simulink model "testConvert2Polyblock"  (Simulink 7.4)
settings: Solver=ode45  StartTime=0.0  StopTime=10.0  RelTol=1e-3
undefined symbols (not defined in the file or in its folder): magnitude
libraries: BLOM_Lib x3
settings Model: Creator=Kyle  LastModifiedBy=Kyle

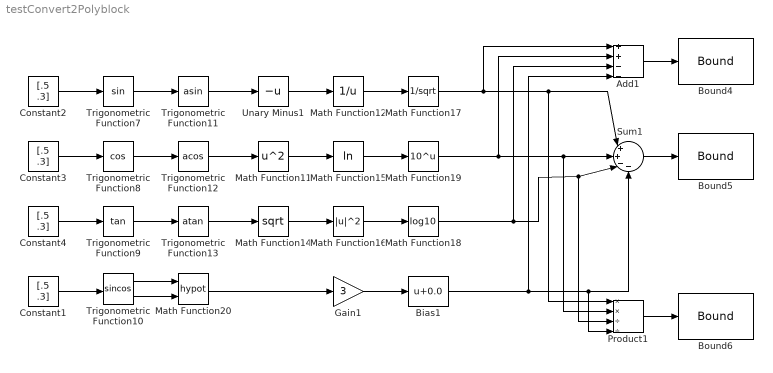
== system testConvert2Polyblock ==
  Add1 : Sum  Inputs=++--  OutDataType=fixdt(1, 16)  OutScaling=2^-10
  Bias1 : Bias  Bias=0.0
  Bound4 : BLOM_Lib/Bound  SystemSampleTime=-1  ub=6  lb=-6  initial_step=on  final_step=off  intermediate_step=off
  Bound5 : BLOM_Lib/Bound  SystemSampleTime=-1  ub=6  lb=-6  initial_step=off  final_step=off  intermediate_step=on
  Bound6 : BLOM_Lib/Bound  SystemSampleTime=-1  ub=6  lb=-6  initial_step=off  final_step=on  intermediate_step=off
  Constant{1..4} (4 alike) : Constant  Value=[.5 .3]  OutDataType=fixdt(1, 16)  OutScaling=2^0
  Gain1 : Gain  Gain=3  ParameterDataType=fixdt(1, 16)  ParameterScaling=2^0  OutDataType=fixdt(1, 16)  OutScaling=2^0
  Math Function11 : Math  Operator=square  OutDataType=fixdt(1, 16)  OutScaling=2^0  SaturateOnIntegerOverflow=on
  Math Function12 : Math  Operator=reciprocal  OutDataType=fixdt(1, 16)  OutScaling=2^0  SaturateOnIntegerOverflow=on
  Math Function14 : Math  Operator=sqrt  OutDataType=fixdt(1, 16)  OutScaling=2^0  SaturateOnIntegerOverflow=on
  Math Function15 : Math  Operator=log  OutDataType=fixdt(1, 16)  OutScaling=2^0  SaturateOnIntegerOverflow=on
  Math Function16 : Math  Operator=magnitude^2  OutDataType=fixdt(1, 16)  OutScaling=2^0  SaturateOnIntegerOverflow=on
  Math Function17 : Math  Operator=1/sqrt  OutDataType=fixdt(1, 16)  OutScaling=2^0  SaturateOnIntegerOverflow=on
  Math Function18 : Math  Operator=log10  OutDataType=fixdt(1, 16)  OutScaling=2^0  SaturateOnIntegerOverflow=on
  Math Function19 : Math  Operator=10^u  OutDataType=fixdt(1, 16)  OutScaling=2^0  SaturateOnIntegerOverflow=on
  Math Function20 : Math  Operator=hypot  OutDataType=fixdt(1, 16)  OutScaling=2^0  SaturateOnIntegerOverflow=on
  Product1 : Product  Inputs=**//  OutDataType=fixdt(1, 16)  OutScaling=2^0  RndMeth=Zero
  Sum1 : Sum  Inputs=|++--  OutDataType=fixdt(1, 16)  OutScaling=2^0
  Trigonometric Function10 : Trigonometry  Operator=sincos
  Trigonometric Function11 : Trigonometry  Operator=asin
  Trigonometric Function12 : Trigonometry  Operator=acos
  Trigonometric Function13 : Trigonometry  Operator=atan
  Trigonometric Function7 : Trigonometry
  Trigonometric Function8 : Trigonometry  Operator=cos
  Trigonometric Function9 : Trigonometry  Operator=tan
  Unary Minus1 : UnaryMinus
  wires:
  Constant2/1 -> Trigonometric Function7/1
  Constant3/1 -> Trigonometric Function8/1
  Constant4/1 -> Trigonometric Function9/1
  Constant1/1 -> Trigonometric Function10/1
  Trigonometric Function7/1 -> Trigonometric Function11/1
  Trigonometric Function8/1 -> Trigonometric Function12/1
  Trigonometric Function9/1 -> Trigonometric Function13/1
  Trigonometric Function11/1 -> Unary Minus1/1
  Trigonometric Function12/1 -> Math Function11/1
  Trigonometric Function10/1 -> Math Function20/1
  Trigonometric Function10/2 -> Math Function20/2
  Trigonometric Function13/1 -> Math Function14/1
  Math Function14/1 -> Math Function16/1
  Unary Minus1/1 -> Math Function12/1
  Math Function12/1 -> Math Function17/1
  Math Function11/1 -> Math Function15/1
  Math Function15/1 -> Math Function19/1
  Math Function16/1 -> Math Function18/1
  Math Function17/1 -> Add1/1, Sum1/1, Product1/1
  Math Function19/1 -> Add1/2, Sum1/2, Product1/2
  Math Function18/1 -> Add1/3, Sum1/3, Product1/3
  Gain1/1 -> Bias1/1
  Bias1/1 -> Add1/4, Sum1/4, Product1/4
  Add1/1 -> Bound4/1
  Sum1/1 -> Bound5/1
  Product1/1 -> Bound6/1
  Math Function20/1 -> Gain1/1
